simulink subsystem "s0330_switching_policy"  (R2019b)
settings: Solver=VariableStepAuto  StartTime=0.0  StopTime=10.0  RelTol=1e-3
settings Model: Creator=paolo  LastModifiedBy=Student

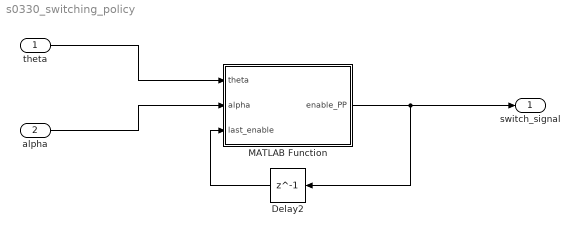
== system s0330_switching_policy ==
  theta : Inport
  alpha : Inport  Port=2
  Delay2 : Delay  DelayLength=1  InitialCondition=false
  MATLAB Function : MATLAB Function  TreatAsAtomicUnit=on
  switch_signal : Outport
  wires:
  theta/1 -> MATLAB Function/1(theta)
  alpha/1 -> MATLAB Function/2(alpha)
  MATLAB Function/1(enable_PP) -> Delay2/1, switch_signal/1
  Delay2/1 -> MATLAB Function/3(last_enable)

== matlab function s0330_switching_policy/MATLAB Function ==
  data: theta input; enable_PP output; alpha input; last_enable input boolean
function enable_PP = PP_enabler(theta, alpha, last_enable)

alpha_diff = alpha*180/pi - 180;
theta = theta*180/pi;

stop_condition = false;
while ~stop_condition
    if alpha_diff > 180
        alpha_diff = alpha_diff - 360;
    elseif alpha_diff < -180
        alpha_diff = alpha_diff + 360;
    else
        stop_condition = true;
    end
end

if (abs(alpha_diff) < 20 && abs(theta) < 200) || last_enable
    enable_PP = true;
else
    enable_PP = false;
end

end
